simulink model "reset"  (R2015b)
settings: Solver=VariableStepAuto  StartTime=0.0  StopTime=10.0  RelTol=1e-3
settings Model: Creator=ladmin  LastModifiedBy=ladmin

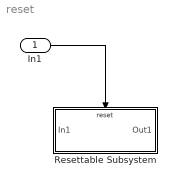
== system reset ==
  In1 : Inport
  Resettable Subsystem : Subsystem  TreatAsAtomicUnit=on
  wires:
  In1/1 -> Resettable Subsystem/Reset

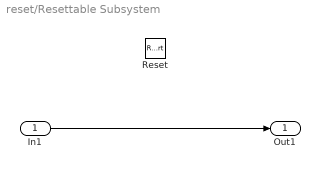
== system reset/Resettable Subsystem ==
  In1 : Inport
  Reset : ResetPort  DisableCoverage=on
  Out1 : Outport
  wires:
  In1/1 -> Out1/1
